simulink model "RedAsociativa"  (Simulink 7.5)
settings: Solver=ode45  StartTime=0.0  StopTime=10.0  RelTol=1e-3
settings Model: Creator=My Laptop  LastModifiedBy=My Laptop

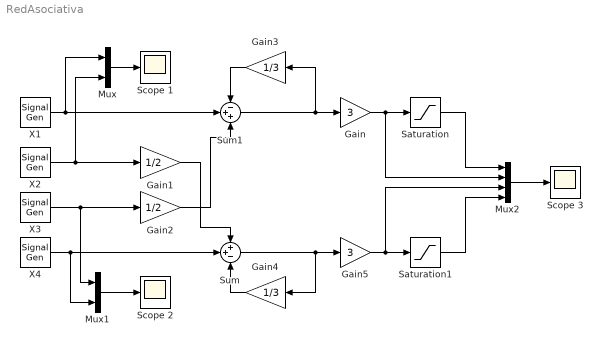
== system RedAsociativa ==
  Gain : Gain  Gain=3  ParameterDataType=fixdt(1, 16)  ParameterScaling=2^0  OutDataType=fixdt(1, 16)  OutScaling=2^0
  Gain1 : Gain  Gain=1/2  ParameterDataType=fixdt(1, 16)  ParameterScaling=2^0  OutDataType=fixdt(1, 16)  OutScaling=2^0
  Gain2 : Gain  Gain=1/2  ParameterDataType=fixdt(1, 16)  ParameterScaling=2^0  OutDataType=fixdt(1, 16)  OutScaling=2^0
  Gain3 : Gain  Gain=1/3  ParameterDataType=fixdt(1, 16)  ParameterScaling=2^0  OutDataType=fixdt(1, 16)  OutScaling=2^0
  Gain4 : Gain  Gain=1/3  ParameterDataType=fixdt(1, 16)  ParameterScaling=2^0  OutDataType=fixdt(1, 16)  OutScaling=2^0
  Gain5 : Gain  Gain=3  ParameterDataType=fixdt(1, 16)  ParameterScaling=2^0  OutDataType=fixdt(1, 16)  OutScaling=2^0
  Mux : Mux  Inputs=2
  Mux1 : Mux  Inputs=2
  Mux2 : Mux
  Saturation : Saturate  UpperLimit=1  LowerLimit=-1  ZeroCross=off  OutDataType=fixdt(1, 16)  OutScaling=2^0
  Saturation1 : Saturate  UpperLimit=1  LowerLimit=-1  ZeroCross=off  OutDataType=fixdt(1, 16)  OutScaling=2^0
  Scope 1 : Scope
      settings: YMin=-1.5  YMax=1.5
  Scope 2 : Scope
      settings: YMin=-1.5  YMax=1.5
  Scope 3 : Scope
      settings: YMin=-1.5  YMax=1.5  SaveName=ScopeData2
  Sum : Sum  Inputs=++-  OutDataType=fixdt(1, 16)  OutScaling=2^0
  Sum1 : Sum  Inputs=-++  OutDataType=fixdt(1, 16)  OutScaling=2^0
  X1 : SignalGenerator  WaveForm=square  Frequency=.8
  X2 : SignalGenerator  WaveForm=square  Frequency=.4
  X3 : SignalGenerator  WaveForm=square  Frequency=.2
  X4 : SignalGenerator  WaveForm=square  Frequency=.1
  wires:
  Mux/1 -> Scope 1/1
  X1/1 -> Mux/1, Sum1/2
  X2/1 -> Mux/2, Gain1/1
  Mux1/1 -> Scope 2/1
  X3/1 -> Mux1/1, Gain2/1
  X4/1 -> Mux1/2, Sum/2
  Gain3/1 -> Sum1/1
  Sum1/1 -> Gain3/1, Gain/1
  Gain4/1 -> Sum/3
  Sum/1 -> Gain4/1, Gain5/1
  Gain2/1 -> Sum1/3
  Gain1/1 -> Sum/1
  Mux2/1 -> Scope 3/1
  Gain/1 -> Saturation/1, Mux2/2
  Gain5/1 -> Saturation1/1, Mux2/3
  Saturation/1 -> Mux2/1
  Saturation1/1 -> Mux2/4
